simulink model "SimCHinf"  (Simulink 10.2)
settings: Solver=ode45  StartTime=0.0  StopTime=100  FixedStep=0.01  MaxStep=0.01  RelTol=1e-3  EnableMultiTasking=on
undefined symbols (not defined in the file): B, J, K1, Ke, Kt, Ra
settings Model: Creator=Harryth  LastModifiedBy=andre
settings DataIOCC: LimitDataPoints=on
settings OptimizationCC: ExpressionDepthLimit=2147483647
settings DebuggingCC: SolverPrmCheckMsg=warning  StateNameClashWarn=warning

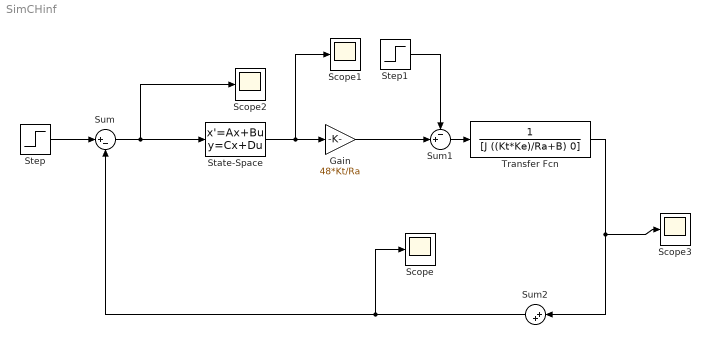
== system SimCHinf ==
  Gain : Gain  Gain=48*Kt/Ra
  Scope{,1..3} (4 alike) : Scope
  State-Space : StateSpace  A=K1.a  B=K1.b  C=K1.c  D=K1.d  InitialCondition=0
  Step : Step  SampleTime=0
  Step1 : Step  Time=5  SampleTime=0
  Sum : Sum  Inputs=|+-
  Sum1 : Sum  Inputs=-+|
  Sum2 : Sum  Inputs=|++
  Transfer Fcn : TransferFcn  Numerator=1  Denominator=[J ((Kt*Ke)/Ra+B) 0]
  wires:
  Step/1 -> Sum/1
  Sum/1 -> Scope2/1, State-Space/1
  Gain/1 -> Sum1/2
  Sum1/1 -> Transfer Fcn/1
  Sum2/1 -> Sum/2, Scope/1
  Transfer Fcn/1 -> Sum2/1, Scope3/1
  Step1/1 -> Sum1/1
  State-Space/1 -> Gain/1, Scope1/1
